simulink model "CH7_2"  (Simulink 5.0)
settings: Solver=ode23tb  StartTime=0.0  StopTime=8/60  MaxStep=1e-5  RelTol=1e-5  AbsTol=1e-5
libraries: powerlib2 x15, powerlib_extras x6, simulink_extras x1
Description:
  | 高苑科技大學 電機系
  | 電力電子實驗室
settings Model: Creator=徐瑞隆老師  LastModifiedBy=ELECTRONIC

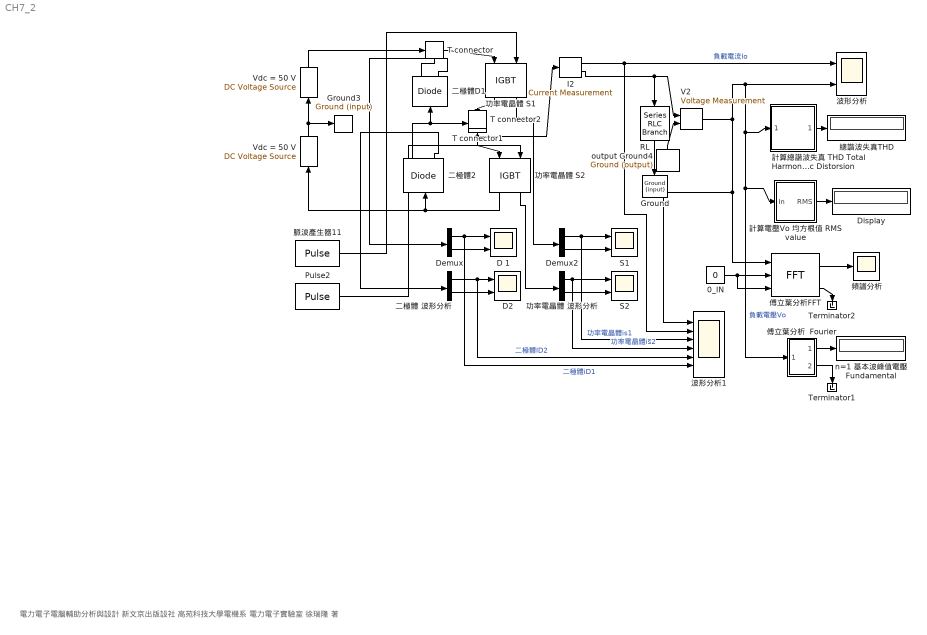
== system CH7_2 ==
  note: 電力電子電腦輔助分析與設計  新文京出版設社
      | 高苑科技大學電機系
      | 電力電子實驗室
      | 徐瑞隆 著
  "   功率電晶體 S2" : powerlib2/Power Electronics/IGBT  Tag=PoWeRsYsTeMbLoCk  Orientation=down  Ron=0.01  Lon=1e-6  Vf=0  Tf=1e-6  Tt=1e-6  IC=0  Rs=10000  Cs=inf  PSBOutputType=10
  0_IN : Constant  Value=0
  D 1 : Scope  NumInputPorts=2
      settings: TimeRange=0.1  YMin=0~-5  YMax=20~5  SaveName=V2X  DataFormat=Array  SampleInput=on  SampleTime=10e-6
  D2 : Scope  NumInputPorts=2
      settings: TimeRange=0.1  YMin=0~-5  YMax=20~5  SaveName=V2X1  DataFormat=Array  SampleInput=on  SampleTime=10e-6
  Demux : Demux  Outputs=2
  Demux2 : Demux  Outputs=2
  Display : Display
  Ground : powerlib2/Connectors/Ground (input)  Tag=PoWeRsYsTeMbLoCk  Orientation=down
  Ground3 : powerlib2/Connectors/Ground (input)  Tag=PoWeRsYsTeMbLoCk
  I2 : powerlib2/Measurements/Current Measurement  Tag=PoWeRsYsTeMmEaSuReMeNt  PhasorSimulation=off  OutputType=Magnitude  PSBOutputType=01  PSBequivalent=0
  Pulse2 : DiscretePulseGenerator  PulseType=Time based  Period=1/60  PulseWidth=50  PhaseDelay=1/120
  "RL   " : powerlib2/Elements/Series RLC Branch  Tag=PoWeRsYsTeMbLoCk  Orientation=down  a=10  b=50e-03  c=inf  mesure=None  PSBOutputType=1
  S1 : Scope  NumInputPorts=2
      settings: TimeRange=0.1  YMin=0~-5  YMax=20~5  SaveName=V2X2  DataFormat=Array  SampleInput=on  SampleTime=10e-6
  S2 : Scope  NumInputPorts=2
      settings: TimeRange=0.1  YMin=0~-5  YMax=20~5  SaveName=V2X3  DataFormat=Array  SampleInput=on  SampleTime=10e-6
  T connector : powerlib2/Connectors/T connector  Tag=PoWeRsYsTeMbLoCk  PSBOutputType=1
  T connector1 : powerlib2/Connectors/T connector  Tag=PoWeRsYsTeMbLoCk  Orientation=down  PSBOutputType=1
  T connector2 : powerlib2/Connectors/T connector  Tag=PoWeRsYsTeMbLoCk  Orientation=down  PSBOutputType=1
  Terminator1 : Terminator
      settings: Orientation=down
  Terminator2 : Terminator
      settings: Orientation=down
  V2 : powerlib2/Measurements/Voltage Measurement  Tag=PoWeRsYsTeMmEaSuReMeNt  PhasorSimulation=off  OutputType=Magnitude  PSBOutputType=0  PSBequivalent=0
  Vdc = 50 V : powerlib2/Electrical Sources/DC Voltage Source  Tag=PoWeRsYsTeMbLoCk  Orientation=up  V=50  mesure=None  PSBOutputType=1
  "Vdc = 50 V " : powerlib2/Electrical Sources/DC Voltage Source  Tag=PoWeRsYsTeMbLoCk  Orientation=up  V=50  mesure=None  PSBOutputType=1
  n=1 基本波峰值電壓 Fundamental : Display
  output Ground4 : powerlib2/Connectors/Ground (output)  Tag=PoWeRsYsTeMbLoCk  Orientation=up  PSBOutputType=1
  二極體 波形分析 : Demux  Outputs=2
  二極體2 : powerlib2/Power Electronics/Diode  Tag=PoWeRsYsTeMbLoCk  Orientation=up  Ron=0.01  Lon=0  Vf=0.8  IC=0  Rs=10  Cs=0.01e-6  PSBOutputType=10
  二極體D1 : powerlib2/Power Electronics/Diode  Tag=PoWeRsYsTeMbLoCk  Orientation=up  Ron=0.01  Lon=0  Vf=0.8  IC=0  Rs=10  Cs=0.01e-6  PSBOutputType=10
  功率電晶體 S1 : powerlib2/Power Electronics/IGBT  Tag=PoWeRsYsTeMbLoCk  Orientation=down  Ron=0.01  Lon=1e-6  Vf=0  Tf=1e-6  Tt=1e-6  IC=0  Rs=10000  Cs=inf  PSBOutputType=10
  "功率電晶體 波形分析 " : Demux  Outputs=2
  波形分析 : Scope  NumInputPorts=2
      settings: TimeRange=0.0333333  YMin=-22.5~-350  YMax=22.5~350  SaveName=psb1phPWM2_str
  波形分析1 : Scope  NumInputPorts=6
      settings: TimeRange=0.0333333  YMin=-22.5~-350~-5~-5~-5~-5  YMax=22.5~350~5~5~5~5  SaveName=psb1phPWM2_str1  MaxDataPoints=30000
  計算電壓Vo 均方根值 RMS value : Subsystem  AncestorBlock=|  mask(Discrete RMS value){Freq=60, Mag_Init=0, Ts=50e-6}
      | powerlib_extras/Discrete
      | Measurements/Discrete 
      | RMS value
      mask prompts: Freq "Fundamental frequency (Hz):"; Mag_Init "Initial magnitude of input:"; Ts "Sample time:"
      mask help:
      | This discrete block measures the root mean square value of instantaneous current or voltage signal connected to the input of the block. The RMS value is calculated over a running window of one cycle of the specified fundamental frequency.
      | For the first cycle of simulation, the ouput is held constant to the RMS value of the specified magnitude of initial input.
  計算總諧波失真 THD Total  Harmonic Distorsion : Subsystem  AncestorBlock=|  mask(Discret Total Harmonic Distortion ){Freq=60, Ts=50e-6}
      | powerlib_extras/Discrete
      | Measurements/Discrete 
      | Total  Harmonic
      | Distorsion
      mask prompts: Freq "Fundamental frequency (Hz):"; Ts "Sample time:"
      mask help:
      | This discrete block measures the total harmonic distortion  (THD ) of a periodic instantaneous voltage or current connected to the input.
      | The THD is defined as:
      |
      |                   THD = Uh/U1
      | where:
      |    Uh = rms value of the harmonics
      |          = sqrt(U2^2 + U3^2 + ....+ Un^2 +...)
      |    U1 = rms value of the fundamental component
  脈波產生器11 : DiscretePulseGenerator  PulseType=Time based  Period=1/60  PulseWidth=50
  傅立葉分析  Fourier : Subsystem  AncestorBlock=|  mask(Discrete Fourier){Freq=60, n=1, Par_Init=[0 0], Ts=50e-6}
      | powerlib_extras/Discrete
      | Measurements/Discrete 
      | Fourier
      mask prompts: Freq "Fundamental frequency (Hz):"; n "Harmonic n (0=DC; 1=fundamental; 2=2nd harm;  ...):"; Par_Init "Initial input: [ Mag  Phase(degrees) ]"; Ts "Sample time:"
      mask help:
      | This block computes the fundamental value of the input signal over a running window of one cycle of the specified fundamental frequency. First and second outputs return respectively the magnitude and phase (degrees) of the fundamental.
      | For the first cycle of simulation, the ouputs are held constant to the value specified by the parameter "Initial input".
      mask init:
      | k=2-(n==0);
      | SamplesPerCycle=1/Freq/Ts;
      | RoundSamplesPerCycle=round(SamplesPerCycle);
      | Delay=RoundSamplesPerCycle*Ts - Ts/2;
      | Correction=SamplesPerCycle/RoundSamplesPerCycle - 1;
      | Real_Init=Par_Init(1)*cos(pi/180*Par_Init(2));
      | Imag_Init=Par_Init(1)*sin(pi/180*Par_Init(2));
  傅立葉分析FFT : powerlib_extras/Discrete Measurements/FFT  f1=60  Ts=200e-6  TsFFT=0.1  base="[1 1  1]"  nDec=0  mask=[1 -1 1]  figure_N=1
  頻譜分析 : Scope
      settings: SaveName=ScopeData2
  總諧波失真THD : Display
  wires:
  Pulse2/1 -> "   功率電晶體 S2"/2
  脈波產生器11/1 -> 功率電晶體 S1/2
  I2/1 -> 波形分析/1, 波形分析1/2  "負載電流Io"
  V2/1 -> 波形分析/2, 計算總諧波失真 THD Total  Harmonic Distorsion/1(signal), 計算電壓Vo 均方根值 RMS value/1(In), 傅立葉分析  Fourier/1(In), 傅立葉分析FFT/1, 波形分析1/1  "負載電壓Vo"
  I2/2 -> "RL   "/1, V2/1
  "Vdc = 50 V "/1 -> Vdc = 50 V/1, Ground3/1
  "RL   "/1 -> Ground/1
  output Ground4/1 -> V2/2
  "   功率電晶體 S2"/1 -> "Vdc = 50 V "/1, 二極體2/1
  T connector/1 -> 功率電晶體 S1/1
  二極體D1/1 -> T connector/Enable
  Vdc = 50 V/1 -> T connector/1
  功率電晶體 S1/1 -> T connector1/1
  T connector1/1 -> "   功率電晶體 S2"/1, I2/1
  二極體2/1 -> T connector1/Enable, 二極體D1/1
  二極體D1/2 -> Demux/1
  二極體2/2 -> 二極體 波形分析/1
  計算電壓Vo 均方根值 RMS value/1(RMS) -> Display/1
  傅立葉分析  Fourier/1(Mag) -> n=1 基本波峰值電壓 Fundamental/1
  傅立葉分析FFT/1 -> 頻譜分析/1
  計算總諧波失真 THD Total  Harmonic Distorsion/1(THD) -> 總諧波失真THD/1
  Demux/1 -> D 1/1, 波形分析1/6  "二極體iD1"
  Demux/2 -> D 1/2
  二極體 波形分析/1 -> D2/1, 波形分析1/5  "二極體ID2"
  二極體 波形分析/2 -> D2/2
  功率電晶體 S1/2 -> Demux2/1
  傅立葉分析FFT/2 -> Terminator2/1
  "   功率電晶體 S2"/2 -> "功率電晶體 波形分析 "/1
  Demux2/1 -> S1/1, 波形分析1/3  "功率電晶體is1"
  Demux2/2 -> S1/2
  "功率電晶體 波形分析 "/1 -> S2/1, 波形分析1/4  "功率電晶體is2"
  "功率電晶體 波形分析 "/2 -> S2/2
  0_IN/1 -> 傅立葉分析FFT/2, 傅立葉分析FFT/3
  傅立葉分析  Fourier/2(Phase) -> Terminator1/1

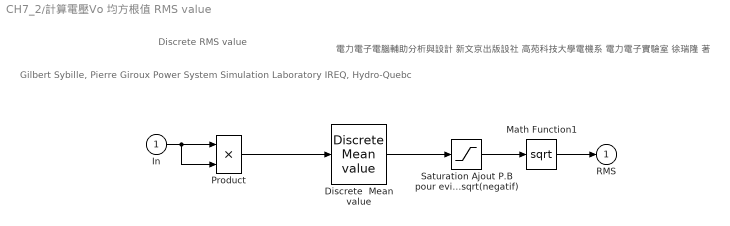
== system CH7_2/計算電壓Vo 均方根值 RMS value ==
  note: Discrete RMS value
  note: Gilbert Sybille, Pierre Giroux
      | Power System Simulation Laboratory
      | IREQ, Hydro-Quebc
  note: 電力電子電腦輔助分析與設計  新文京出版設社
      | 高苑科技大學電機系
      | 電力電子實驗室
      | 徐瑞隆 著
  In : Inport
  Discrete  Mean value : powerlib_extras/Discrete Measurements/Discrete  Mean value  AncestorBlock=|  Freq=Freq  Vinit=sqrt(Mag_Init)  Ts=Ts
      | powerlib_extras/Discrete
      | Measurements/Discrete 
      | Mean value
  Math Function1 : Math  Operator=sqrt
  Product : Product  SaturateOnIntegerOverflow=on  InputSameDT=on
  Saturation Ajout P.B pour eviter  sqrt(negatif) : Saturate  UpperLimit=Inf  LowerLimit=0
  RMS : Outport  InitialOutput=0
  wires:
  Saturation Ajout P.B pour eviter  sqrt(negatif)/1 -> Math Function1/1
  Discrete  Mean value/1 -> Saturation Ajout P.B pour eviter  sqrt(negatif)/1
  Product/1 -> Discrete  Mean value/1
  Math Function1/1 -> RMS/1
  In/1 -> Product/1, Product/2

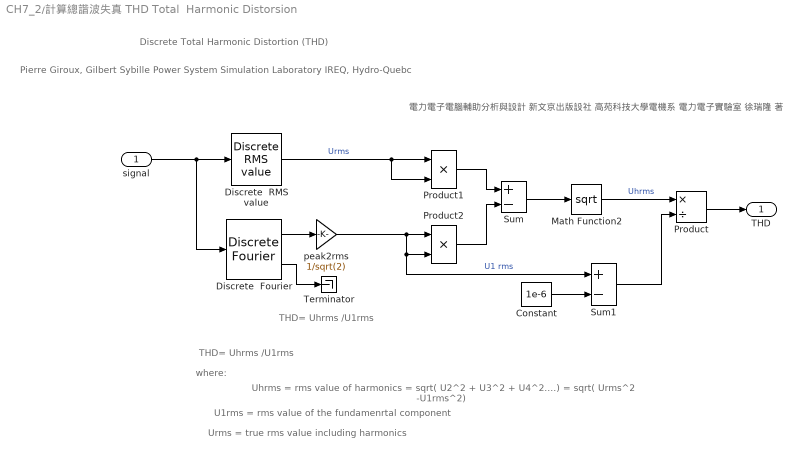
== system CH7_2/計算總諧波失真 THD Total  Harmonic Distorsion ==
  note: THD= Uhrms /U1rms
  note: where:
  note: U1rms = rms value of the fundamenrtal component
  note: Uhrms = rms value of harmonics = sqrt( U2^2 + U3^2 + U4^2....) = sqrt( Urms^2 -U1rms^2)
  note: Urms = true rms value including harmonics
  note: THD= Uhrms /U1rms
  note: Discrete Total Harmonic Distortion (THD)
  note: Pierre Giroux, Gilbert Sybille
      | Power System Simulation Laboratory
      | IREQ, Hydro-Quebc
  note: 電力電子電腦輔助分析與設計  新文京出版設社
      | 高苑科技大學電機系
      | 電力電子實驗室
      | 徐瑞隆 著
  signal : Inport
  Constant : Constant  Value=1e-6
  Discrete  Fourier : powerlib_extras/Discrete Measurements/Discrete  Fourier  Freq=Freq  n=1  Par_Init=[0 0]  Ts=Ts
  Discrete  RMS value : powerlib_extras/Discrete Measurements/Discrete  RMS value  Freq=Freq  Mag_Init=0  Ts=Ts
  Math Function2 : Math  Operator=sqrt
  Product : Product  Inputs=*/  SaturateOnIntegerOverflow=on  InputSameDT=on
  Product1 : Product  SaturateOnIntegerOverflow=on  InputSameDT=on
  Product2 : Product  SaturateOnIntegerOverflow=on  InputSameDT=on
  Sum : Sum  Inputs=+-  SaturateOnIntegerOverflow=on  InputSameDT=on
  Sum1 : Sum  Inputs=+-  SaturateOnIntegerOverflow=on  InputSameDT=on
  Terminator : Terminator
  peak2rms : Gain  Gain=1/sqrt(2)  SaturateOnIntegerOverflow=on
  THD : Outport
  wires:
  Discrete  Fourier/2 -> Terminator/1
  peak2rms/1 -> Product2/1, Sum1/1, Product2/2  "U1 rms"
  Discrete  Fourier/1 -> peak2rms/1
  Product/1 -> THD/1
  Math Function2/1 -> Product/1  "Uhrms"
  Product2/1 -> Sum/2
  Product1/1 -> Sum/1
  Sum/1 -> Math Function2/1
  signal/1 -> Discrete  RMS value/1, Discrete  Fourier/1
  Discrete  RMS value/1 -> Product1/1, Product1/2  "Urms"
  Constant/1 -> Sum1/2
  Sum1/1 -> Product/2

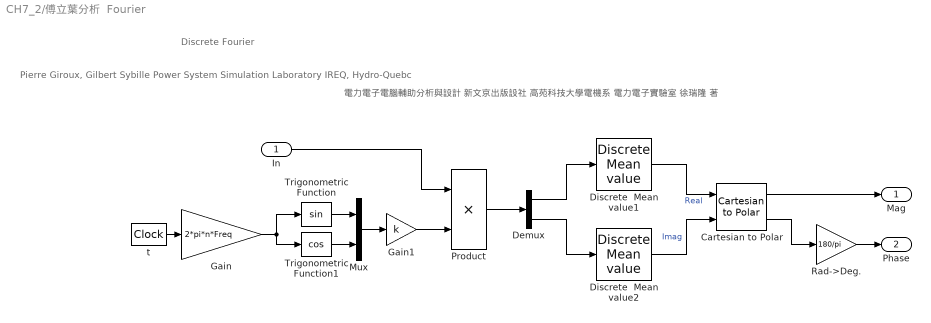
== system CH7_2/傅立葉分析  Fourier ==
  note: Pierre Giroux, Gilbert Sybille
      | Power System Simulation Laboratory
      | IREQ, Hydro-Quebc
  note: Discrete Fourier
  note: 電力電子電腦輔助分析與設計  新文京出版設社
      | 高苑科技大學電機系
      | 電力電子實驗室
      | 徐瑞隆 著
  In : Inport
  Cartesian to Polar : simulink_extras/Transformations/Cartesian to Polar
  Demux : Demux  Outputs=2
  Discrete  Mean value1 : powerlib_extras/Discrete Measurements/Discrete  Mean value  AncestorBlock=|  Freq=Freq  Vinit=Real_Init  Ts=Ts
      | powerlib_extras/Discrete
      | Measurements/Discrete 
      | Mean value
  Discrete  Mean value2 : powerlib_extras/Discrete Measurements/Discrete  Mean value  AncestorBlock=|  Freq=Freq  Vinit=Imag_Init  Ts=Ts
      | powerlib_extras/Discrete
      | Measurements/Discrete 
      | Mean value
  Gain : Gain  Gain=2*pi*n*Freq  SaturateOnIntegerOverflow=on
  Gain1 : Gain  Gain=k  SaturateOnIntegerOverflow=on
  Mux : Mux  Inputs=2
  Product : Product  SaturateOnIntegerOverflow=on  InputSameDT=on
  Rad->Deg. : Gain  Gain=180/pi  SaturateOnIntegerOverflow=on
  Trigonometric Function : Trigonometry
  Trigonometric Function1 : Trigonometry  Operator=cos
  t : DigitalClock  SampleTime=Ts
  Mag : Outport
  Phase : Outport  Port=2
  wires:
  Rad->Deg./1 -> Phase/1
  Cartesian to Polar/1 -> Mag/1
  Cartesian to Polar/2 -> Rad->Deg./1
  Discrete  Mean value2/1 -> Cartesian to Polar/2  "Imag"
  Discrete  Mean value1/1 -> Cartesian to Polar/1  "Real"
  Demux/2 -> Discrete  Mean value2/1
  Demux/1 -> Discrete  Mean value1/1
  Product/1 -> Demux/1
  Gain1/1 -> Product/2
  In/1 -> Product/1
  Mux/1 -> Gain1/1
  Trigonometric Function1/1 -> Mux/2
  Trigonometric Function/1 -> Mux/1
  Gain/1 -> Trigonometric Function1/1, Trigonometric Function/1
  t/1 -> Gain/1
